simulink model "pid_design_final"  (R2019b)
settings: Solver=ode1  StartTime=0.0  StopTime=10  FixedStep=0.001  RelTol=1e-3
settings Model: DataTypeOverride=Double  MinMaxOverflowLogging=ForceOff  Creator=subhgang  LastModifiedBy=subhgang

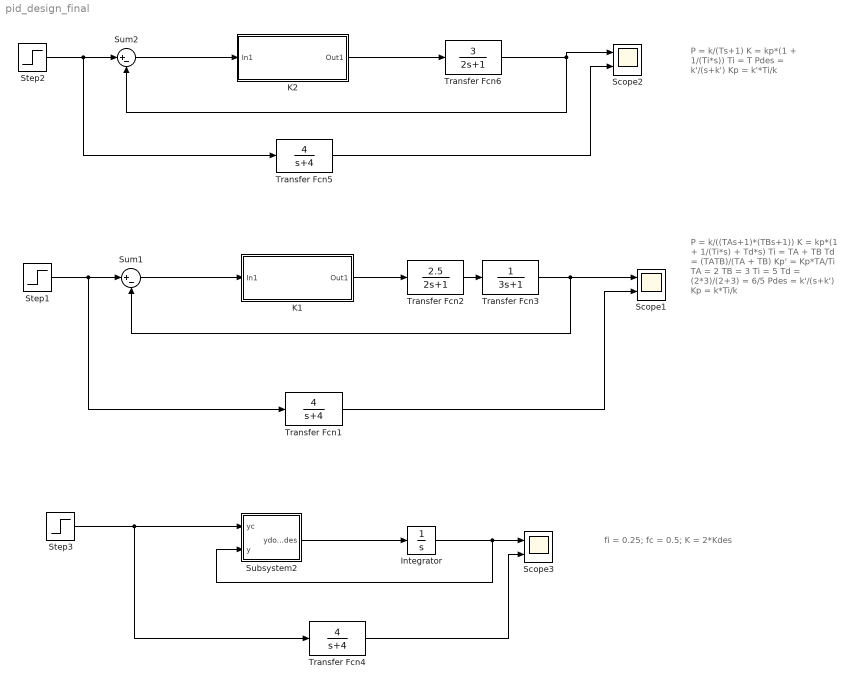
== system pid_design_final ==
  note: fi = 0.25;
      | fc = 0.5;
      | K = 2*Kdes
  note: P = k/((TAs+1)*(TBs+1))
      |
      | K = kp*(1 + 1/(Ti*s) + Td*s)
      |
      | Ti = TA + TB
      | Td = (TATB)/(TA + TB)
      | Kp' = Kp*TA/Ti
      |
      | TA = 2
      | TB = 3
      |
      | Ti = 5
      | Td = (2*3)/(2+3) = 6/5
      |
      | Pdes = k'/(s+k')
      |
      | Kp = k*Ti/k
  note: P = k/(Ts+1)
      |
      | K = kp*(1 + 1/(Ti*s))
      |
      | Ti = T
      |
      | Pdes = k'/(s+k')
      |
      | Kp = k'*Ti/k
  Integrator : Integrator
  K1 : Subsystem
  K2 : Subsystem
  Scope1 : Scope  NumInputPorts=2
  Scope2 : Scope  NumInputPorts=2
  Scope3 : Scope  NumInputPorts=2
  Step1 : Step  SampleTime=0
  Step2 : Step  SampleTime=0
  Step3 : Step  SampleTime=0
  Subsystem2 : Subsystem
  Sum1 : Sum  Inputs=|+-
  Sum2 : Sum  Inputs=|+-
  Transfer Fcn1 : TransferFcn  Numerator=[4]  Denominator=[1 4]
  Transfer Fcn2 : TransferFcn  Numerator=[2.5]  Denominator=[2 1]
  Transfer Fcn3 : TransferFcn  Denominator=[3 1]
  Transfer Fcn4 : TransferFcn  Numerator=[4]  Denominator=[1 4]
  Transfer Fcn5 : TransferFcn  Numerator=[4]  Denominator=[1 4]
  Transfer Fcn6 : TransferFcn  Numerator=[3]  Denominator=[2 1]
  wires:
  K1/1(Out1) -> Transfer Fcn2/1
  Step1/1 -> Transfer Fcn1/1, Sum1/1
  Transfer Fcn2/1 -> Transfer Fcn3/1
  Sum1/1 -> K1/1(In1)
  Transfer Fcn1/1 -> Scope1/2
  Transfer Fcn3/1 -> Scope1/1, Sum1/2
  K2/1(Out1) -> Transfer Fcn6/1
  Step2/1 -> Transfer Fcn5/1, Sum2/1
  Transfer Fcn6/1 -> Scope2/1, Sum2/2
  Sum2/1 -> K2/1(In1)
  Transfer Fcn5/1 -> Scope2/2
  Integrator/1 -> Subsystem2/2(y), Scope3/1
  Step3/1 -> Subsystem2/1(yc), Transfer Fcn4/1
  Transfer Fcn4/1 -> Scope3/2
  Subsystem2/1(ydot_des) -> Integrator/1

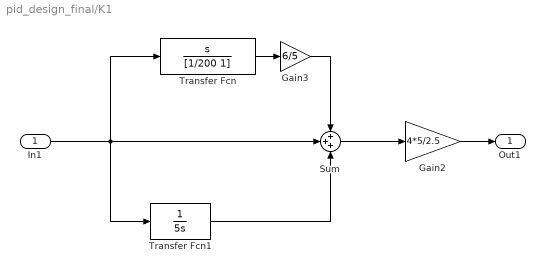
== system pid_design_final/K1 ==
  In1 : Inport
  Gain2 : Gain  Gain=4*5/2.5
  Gain3 : Gain  Gain=6/5
  Sum : Sum  Inputs=+++
  Transfer Fcn : TransferFcn  Numerator=[1 0]  Denominator=[1/200 1]
  Transfer Fcn1 : TransferFcn  Denominator=[5 0]
  Out1 : Outport
  wires:
  Sum/1 -> Gain2/1
  Gain2/1 -> Out1/1
  Transfer Fcn/1 -> Gain3/1
  In1/1 -> Transfer Fcn1/1, Sum/2, Transfer Fcn/1
  Transfer Fcn1/1 -> Sum/3
  Gain3/1 -> Sum/1

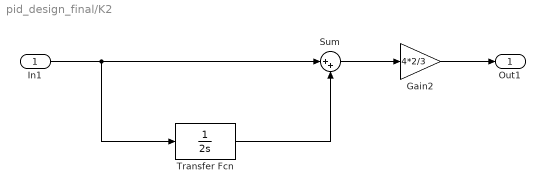
== system pid_design_final/K2 ==
  In1 : Inport
  Gain2 : Gain  Gain=4*2/3
  Sum : Sum  Inputs=|++
  Transfer Fcn : TransferFcn  Denominator=[2 0]
  Out1 : Outport
  wires:
  In1/1 -> Transfer Fcn/1, Sum/1
  Sum/1 -> Gain2/1
  Gain2/1 -> Out1/1
  Transfer Fcn/1 -> Sum/2

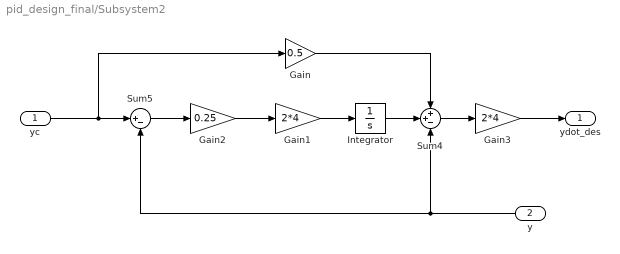
== system pid_design_final/Subsystem2 ==
  yc : Inport
  y : Inport  Port=2
  Gain : Gain  Gain=0.5
  Gain1 : Gain  Gain=2*4
  Gain2 : Gain  Gain=0.25
  Gain3 : Gain  Gain=2*4
  Integrator : Integrator
  Sum4 : Sum  Inputs=++-
  Sum5 : Sum  Inputs=|+-
  ydot_des : Outport  VectorParamsAs1DForOutWhenUnconnected=off
  wires:
  y/1 -> Sum4/3, Sum5/2
  Gain/1 -> Sum4/1
  Integrator/1 -> Sum4/2
  yc/1 -> Sum5/1, Gain/1
  Sum5/1 -> Gain2/1
  Sum4/1 -> Gain3/1
  Gain2/1 -> Gain1/1
  Gain1/1 -> Integrator/1
  Gain3/1 -> ydot_des/1
